simulink model "filter_bank_test"  (R2019b)
settings: Solver=FixedStepDiscrete  StartTime=0.0  StopTime=0.001  FixedStep=1e-6  RelTol=1e-3
undefined symbols (not defined in the file or in its folder): image, port_label
libraries: aldec_ahdl x2, simulink_extras x1, dspsrcs4 x1
settings Model: Creator=thomas  LastModifiedBy=thomas

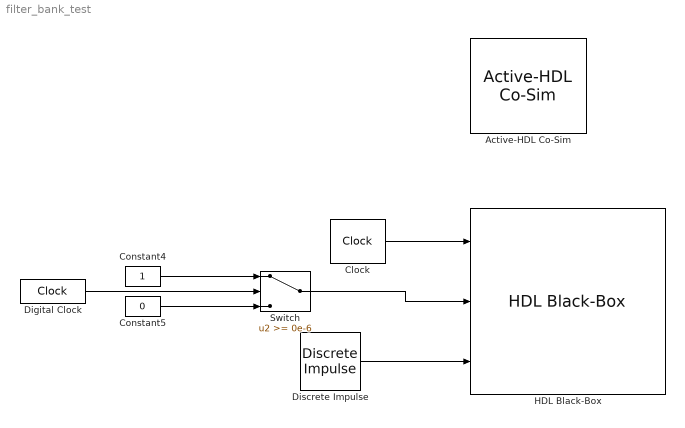
== system filter_bank_test ==
  Active-HDL Co-Sim : aldec_ahdl/Active-HDL Co-Sim  Tag=Active-HDL_Co-Sim_close  hdl_period=1  hdl_tscale=us  sys_period=[1, 0]  sys_tscale=As In Simulator  cmd_after_vsim=wave -noreg -notation 2complement -dec -height 100 {/filter_bank_test/\filter_bank_test/HDL Black-Box\/DOUT}  wav_fn=$(model_name)  wav_settings=[0,3]  sim_cfg=[0,0,0]  dbg=off  auto_start=off  gen_tb=[0,1,15]  batch_sim=off  tb_fn=$(model_name).log  metavalue_map=[0,0]  sim_resolution=[1,0,0]  active_page=2  aws_en=off  ahdl_en=off  blk_ver=10.5a.RTM  macro_en=[0,0,0]
      settings: SourceProductName=Active-HDL Toolbox
  Clock : simulink_extras/Flip Flops/Clock  period=6e-6
  Constant4 : Constant
  Constant5 : Constant  Value=0
  Digital Clock : DigitalClock  SampleTime=1e-6
  Discrete Impulse : dspsrcs4/Discrete  Impulse  Delay=100  SampleTime=6e-6  FrameSample=1  OutputFrames=off  dataType=double  isSigned=on  wordLen=16  udDataType=sfix(16)  fracBitsMode=Best precision  numFracBits=15  OutDataTypeStr=double  LastOutDataTypeStr=double
  HDL Black-Box : aldec_ahdl/HDL Black-Box  Tag=Active-HDL_BB_lib  module_m=filter_bank  ports_cfg={CLK,0,1,2,0,Inherited,8,0,0,0,0,1}{ARESTN,0,1,2,0,Inherited,8,0,0,0,0,1}{DIN,0,-1,2,0,Inherited,0,0,0,0,0,1}{DOUT,1,-1,2,0,1,0,0,0,1,0,0}  params={CHANNELS,32,INTEGER}{OVERSAMPLING_RATE,1,INTEGER}{AXIS_IQ_TDATA_WIDTH,32,INTEGER}  waves={2,Inputs,2,3,0,15,,-1,-1,-1,0,0,0,0}{0,CLK,0,0,0,15,,-1,-1,-1,0,0,0,0}{0,ARESTN,0,0,0,15,,-1,-1,-1,0,0,0,0}{0,DIN,2,2,0,15,,-1,-1,-1,1,0,0,0}{2,Outputs,2,3,0,15,,-1,-1,-1,0,0,0,0}  block_mask=image('HDLBlackBox.jpg','center'); disp('filter_bank');port_label('input', 1, 'CLK');port_label('input', 2, 'ARESTN');port_label('input', 3, 'DIN');  config=[3,0]  inp=[3, 8, 1, 0, 0, 0, 2, 8, 1, 0, 0, 0, 2, 0, abs(32-1 - 0) + 1, 0, 0, 0, 2]  out=[0]  sampling=[1, -1, -1, -1]  active_page={1004,476,5,{0,{80,0,0,1},{35,1,2,1},{65,2,2,1},{70,3,2,1},{70,4,2,1},{60,5,2,1},{60,6,2,1},{50,7,2,1},{35,8,2,1},{35,9,2,1},{119,10,0,1}},{1,{138,0,0,1},{55,1,2,1},{70,2,2,1},{75,3,2,1},{75,4,2,1},{45,5,2,1},{45,6,2,1},{45,7,2,1},{165,8,0,1}},{2,{165,0,0,1},{130,1,2,1},{190,2,2,1},{190,3,2,1}},{3,{94,0,0,1},{58,1,2,1},{58,2,2,1},{70,3,2,1},{58,4,2,1}},{4,{83,0,0,1},{70,1,2,1},{80,2,2,1},{50,3,2,1},{50,4,2,1}},{5,{125,0,0,1},{330,1,2,1},{220,2,2,1}},{6,{95,0,0,1},{95,1,1,1},{70,2,2,1},{50,3,1,1},{80,4,1,1},{35,5,2,1},{35,6,2,1},{65,7,0,1},{150,8,0,1}}}  param_val={32,-1,1,-1,32,-1}  clk_val=[0]  ce_val=[0]  blk_ver=10.5a.RTM  blk_conf=0  user_conv=0
      settings: SourceProductName=Active-HDL Toolbox
  Switch : Switch  Threshold=0e-6
  wires:
  Discrete Impulse/1 -> HDL Black-Box/3
  Digital Clock/1 -> Switch/2
  Constant5/1 -> Switch/3
  Constant4/1 -> Switch/1
  Switch/1 -> HDL Black-Box/2
  Clock/1 -> HDL Black-Box/1
